simulink model "motorisation_energy_chain"  (R2019b)
settings: Solver=VariableStepAuto  StartTime=0.0  StopTime=10.0  RelTol=1e-3
libraries: simulink x2
settings Model: Creator=ZHOU Jinhan  LastModifiedBy=ZHOU Jinhan

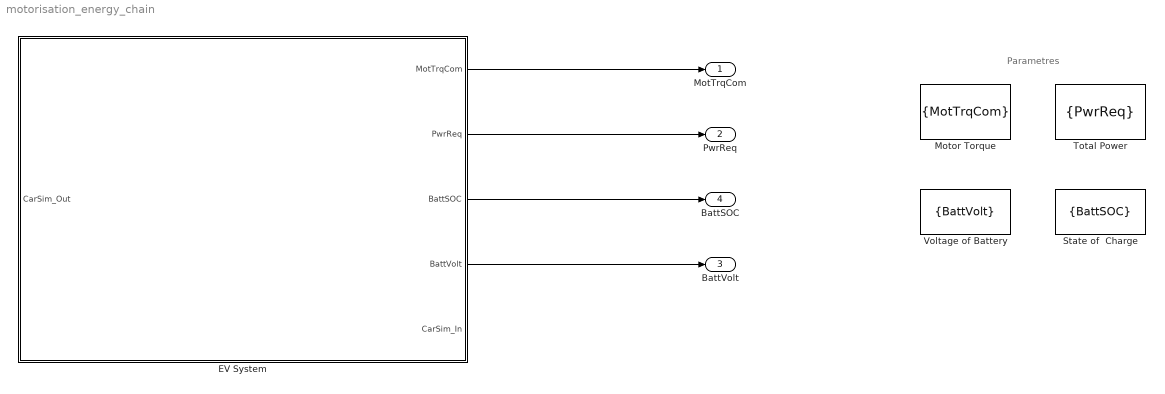
== system motorisation_energy_chain ==
  note: Parametres
  EV System : Subsystem  mask{AmbTem=25, R=0.265}
      mask Display: image('$imagefile'); % Use "Edit Image" on toolstrip to change.
  Motor Torque : GotoTagVisibility  GotoTag=MotTrqCom
  State of  Charge : GotoTagVisibility  GotoTag=BattSOC
  Total Power : GotoTagVisibility  GotoTag=PwrReq
  Voltage of Battery : GotoTagVisibility  GotoTag=BattVolt
  MotTrqCom : Outport
  PwrReq : Outport  Port=2
  BattVolt : Outport  Port=3
  BattSOC : Outport  Port=4
  wires:
  EV System/1(MotTrqCom) -> MotTrqCom/1
  EV System/2(PwrReq) -> PwrReq/1
  EV System/3(BattSOC) -> BattSOC/1
  EV System/4(BattVolt) -> BattVolt/1

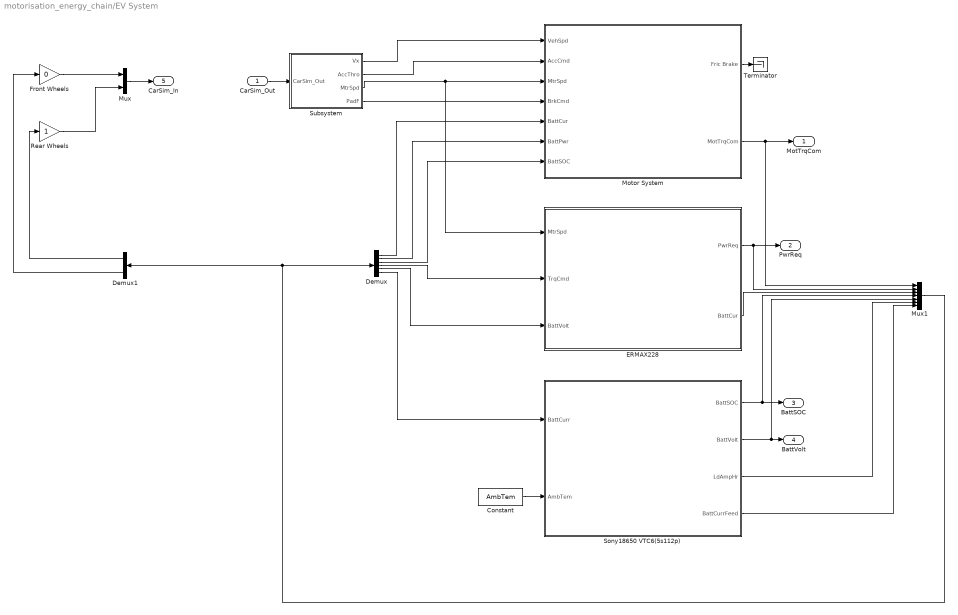
== system motorisation_energy_chain/EV System ==
  CarSim_Out : Inport
  Constant : Constant  Value=AmbTem
  Demux : Demux  Outputs=6
  Demux1 : Demux  Outputs=2
  ERMAX228 : Subsystem  mask{Eff=[83 84 85 84.5 85 84.8 84.59999999999999 84.3 84 83.5 82.8;84 84 86 86 85.8 85.59999999999999 85.59999999999999 85.2 84.5 84 83.3;84 86 87.5 88 88 88 87 86 85 84.5 83.90000000000001;84 87 88.5 90 91 91 90 88 86.2 85.5 84.5;84 87.5 89.5 93.8 93.5 93.8 94.3 91 89.5 86.5 85;84 88 92 94.2 94.5 94.5 95 94 91 91.5 85.8;84 88 92.5 94.59999999999999 95 95.3 95.40000000000001 94.7 92 90.2 85.8;84 88 93 95.59999999999999 96.2 96.3 95.40000000000001 94.90000000000001 93 90.2 85.5;84 88 93 95.8 96.40000000000001 97 95.40000000000001 94.90000000000001 94 90.2 85.8;84 88 92 96 96.59999999999999 97.5 95.40000000000001 94.90000000000001 94 90.2 85.8;84 88 93 95.90000000000001 98 97.5 95.40000000000001 94.90000000000001 94 90.2 85.8;84 88 93 95.90000000000001 97.5 97.5 95.40000000000001 94.90000000000001 94 90.2 85.8;84 88 93 95.59999999999999 97 97.5 95.40000000000001 94.90000000000001 94 90.2 85.8;84 88 93 95.5 96.8 97.3 95.40000000000001 94.90000000000001 94 90.2 85.8;84 86 93 95 96.40000000000001 96.5 95.40000000000001 94.90000000000001 94 90.2 85.8;83.5 85 93 94.8 96.2 96.2 95.40000000000001 94.8 94 90.2 85.8;83.5 84 92 94.59999999999999 95.7 95.7 95.2 94.8 94 90.2 85.8;83.2 83.5 89.5 94.40000000000001 95.2 95.5 95.09999999999999 94.7 94 90.2 85.8;83 83.2 88 94 94.7 95.2 95 94.59999999999999 94 90.2 85.8;82.7 83 86 91 94.3 94.5 94.8 94.59999999999999 94 90.2 85.8;82.5 83.7 85 92 93.8 94.2 94.5 94.5 94 90.2 85.8;82.3 83.40000000000001 84 90 90 93 94.3 94.3 94 90.2 85.8;82 82.7 83 84 85.2 86 94 94 94 90.2 85.8], MtrSpd_sample=[0 1200 1400 1600 1800 2000 2200 2400 2600 2800 3000 3200 3400 3600 3800 4000 4200 4400 4600 4800 5000 6000 7000], MtrTrq_sample=[240 240 240 240 240 240 240 239.1 237.8 236.6 235.7 234.5 233.1 231.6 230.6 228 225.8 222.9 220.6 217.7 216.2 216 216], Spd=[0 250 500 750 1000 1250 1500 1750 2000 2250 2500 2750 3000 3250 3500 3750 4000 4250 4500 4750 5000 5250 5500], Tc=0.02, Trq=[0 25 50 75 100 125 150 175 200 225 250]}
      mask Display: image('$imagefile'); % Use "Edit Image" on toolstrip to change.
  Front Wheels : Gain  Gain=0
  Motor System : Subsystem  mask(DatasheetMotor){Eff=[83 84 85 84.5 85 84.8 84.59999999999999 84.3 84 83.5 82.8;84 84 86 86 85.8 85.59999999999999 85.59999999999999 85.2 84.5 84 83.3;84 86 87.5 88 88 88 87 86 85 84.5 83.90000000000001;84 87 88.5 90 91 91 90 88 86.2 85.5 84.5;84 87.5 89.5 93.8 93.5 93.8 94.3 91 89.5 86.5 85;84 88 92 94.2 94.5 94.5 95 94 91 91.5 85.8;84 88 92.5 94.59999999999999 95 95.3 95.40000000000001 94.7 92 90.2 85.8;84 88 93 95.59999999999999 96.2 96.3 95.40000000000001 94.90000000000001 93 90.2 85.5;84 88 93 95.8 96.40000000000001 97 95.40000000000001 94.90000000000001 94 90.2 85.8;84 88 92 96 96.59999999999999 97.5 95.40000000000001 94.90000000000001 94 90.2 85.8;84 88 93 95.90000000000001 98 97.5 95.40000000000001 94.90000000000001 94 90.2 85.8;84 88 93 95.90000000000001 97.5 97.5 95.40000000000001 94.90000000000001 94 90.2 85.8;84 88 93 95.59999999999999 97 97.5 95.40000000000001 94.90000000000001 94 90.2 85.8;84 88 93 95.5 96.8 97.3 95.40000000000001 94.90000000000001 94 90.2 85.8;84 86 93 95 96.40000000000001 96.5 95.40000000000001 94.90000000000001 94 90.2 85.8;83.5 85 93 94.8 96.2 96.2 95.40000000000001 94.8 94 90.2 85.8;83.5 84 92 94.59999999999999 95.7 95.7 95.2 94.8 94 90.2 85.8;83.2 83.5 89.5 94.40000000000001 95.2 95.5 95.09999999999999 94.7 94 90.2 85.8;83 83.2 88 94 94.7 95.2 95 94.59999999999999 94 90.2 85.8;82.7 83 86 91 94.3 94.5 94.8 94.59999999999999 94 90.2 85.8;82.5 83.7 85 92 93.8 94.2 94.5 94.5 94 90.2 85.8;82.3 83.40000000000001 84 90 90 93 94.3 94.3 94 90.2 85.8;82 82.7 83 84 85.2 86 94 94 94 90.2 85.8], Batt_R1=0.015, MtrSpd_sample=[0 1200 1400 1600 1800 2000 2200 2400 2600 2800 3000 3200 3400 3600 3800 4000 4200 4400 4600 4800 5000 6000 7000], MtrTrq_sample=[240 240 240 240 240 240 240 239.1 237.8 236.6 235.7 234.5 233.1 231.6 230.6 228 225.8 222.9 220.6 217.7 216.2 216 216], Np=5, Ns=112, Pedal_Acc=[0 50 100], Pedal_Spd=[0 250 500 750 1000 1250 1500 1750 2000 2250 2500 2750 3000 3250 3500 3750 4000 4250 4500 4750 5000 5250 5500], Pedal_Trq=[0 0 0 0 0 0 0 0 0 0 0 0 0 0 0 0 0 0 0 0 0 0 0;96 99 102 106 108 112 114 118 120 121 123 126 126 126 126 125 123 120 120 120 115 111 108;240 240 240 240 240 240 240 239.1 237.8 236.6 235.7 234.5 233.1 231.6 230.6 228 225.8 222.9 220.6 217.7 216.2 216 216], PowerLimitBuffer=60000, Power_charge=[89.85599999999999 101.4 102.336 102.96 103.584 104.208 104.52 111.696], Power_discharge=[102.96 102.336 101.4 100.776 100.152 99.84 99.21600000000001 82.67999999999999], SOC_charge=[0 0.15625 0.3125 0.46875 0.625 0.78125 0.9375 1], SOC_discharge=[0 0.15625 0.3125 0.46875 0.625 0.78125 0.9375 1], Spd=[0 250 500 750 1000 1250 1500 1750 2000 2250 2500 2750 3000 3250 3500 3750 4000 4250 4500 4750 5000 5250 5500], Trq=[0 25 50 75 100 125 150 175 200 225 250], Tsb=0.15, Tst=0.1}
      mask Display: image('$imagefile'); % Use "Edit Image" on toolstrip to change.
  Mux : Mux  Inputs=2
  Mux1 : Mux  Inputs=7
  Rear Wheels : Gain
  Sony18650 VTC6(5s112p) : Subsystem  mask{RInt=[18 17 16 15 13 11 10 9.5 9.5 9.5 9.5 9.5;18 16 15 13 11 10 9.5 9 9 9 9 9;18 15 13 11 10 9 8.5 8.5 8.5 8.5 8.5 8.5;18 9 8 8 8 8 8 8 8 8 8 8;18 8 8 8 8 8 8 8 8 8 8 8;18 8 8 8 8 8 8 8 8 8 8 8], BattCapinit=2.85, CapLUTBp=[0 5 10 20 30 40 50 60 70 80 90 100], CapSOCBp=[0 5 10 20 30 40 50 60 70 80 90 100], BattTempBp=[-10 0 10 25 40 45], Em=[3 3.45 3.68 3.74 3.77 3.79 3.82 3.87 3.92 3.98 4.06 4.2], Np=5, Ns=112, CapTem=[-10 0 23 45], CapNom=[2.517894736842106 2.652547368421053 3.120000000000001 3.120000000000001]}
      mask Display: image('$imagefile'); % Use "Edit Image" on toolstrip to change.
  Subsystem : Subsystem
  Terminator : Terminator
  MotTrqCom : Outport
  PwrReq : Outport  Port=2
  BattSOC : Outport  Port=3
  BattVolt : Outport  Port=4
  CarSim_In : Outport  Port=5
  wires:
  Front Wheels/1 -> Mux/1
  Subsystem/1(Vx) -> Motor System/1(VehSpd)
  Sony18650 VTC6(5s112p)/2(BattVolt) -> Mux1/5, BattVolt/1
  Motor System/2(MotTrqCom) -> Mux1/1, MotTrqCom/1
  Subsystem/4(PadF) -> Motor System/4(BrkCmd)
  Motor System/1(Fric Brake) -> Terminator/1
  Subsystem/2(AccThro) -> Motor System/2(AccCmd)
  Subsystem/3(MtrSpd) -> ERMAX228/1(MtrSpd), Motor System/3(MtrSpd)
  ERMAX228/1(PwrReq) -> Mux1/2, PwrReq/1
  Constant/1 -> Sony18650 VTC6(5s112p)/2(AmbTem)
  Sony18650 VTC6(5s112p)/1(BattSOC) -> Mux1/4, BattSOC/1
  CarSim_Out/1 -> Subsystem/1(CarSim_Out)
  Mux/1 -> CarSim_In/1
  Rear Wheels/1 -> Mux/2
  ERMAX228/2(BattCur) -> Mux1/3
  Sony18650 VTC6(5s112p)/3(LdAmpHr) -> Mux1/6
  Sony18650 VTC6(5s112p)/4(BattCurrFeed) -> Mux1/7
  Mux1/1 -> Demux/1, Demux1/1
  Demux/1 -> Motor System/5(BattCur)
  Demux/2 -> Motor System/6(BattPwr)
  Demux/3 -> Motor System/7(BattSOC)
  Demux/4 -> ERMAX228/2(TrqCmd)
  Demux/5 -> ERMAX228/3(BattVolt)
  Demux/6 -> Sony18650 VTC6(5s112p)/1(BattCurr)
  Demux1/1 -> Rear Wheels/1
  Demux1/2 -> Front Wheels/1

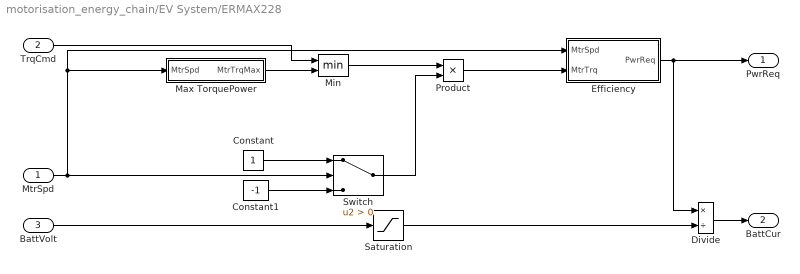
== system motorisation_energy_chain/EV System/ERMAX228 ==
  MtrSpd : Inport
  TrqCmd : Inport  Port=2
  BattVolt : Inport  Port=3
  Constant : Constant
  Constant1 : Constant  Value=-1
  Divide : Product  Inputs=*/
  Efficiency : Subsystem
  Max TorquePower : Subsystem
  Min : MinMax  Inputs=2
  Product : Product
  Saturation : Saturate  UpperLimit=Inf  LowerLimit=0.001
  Switch : Switch  Criteria=u2 > Threshold
  PwrReq : Outport
  BattCur : Outport  Port=2
  wires:
  Saturation/1 -> Divide/2
  BattVolt/1 -> Saturation/1
  Divide/1 -> BattCur/1
  Switch/1 -> Product/2
  TrqCmd/1 -> Min/1
  Max TorquePower/1(MtrTrqMax) -> Min/2
  Product/1 -> Efficiency/2(MtrTrq)
  Min/1 -> Product/1
  Constant/1 -> Switch/1
  Constant1/1 -> Switch/3
  Efficiency/1(PwrReq) -> PwrReq/1, Divide/1
  MtrSpd/1 -> Switch/2, Max TorquePower/1(MtrSpd), Efficiency/1(MtrSpd)

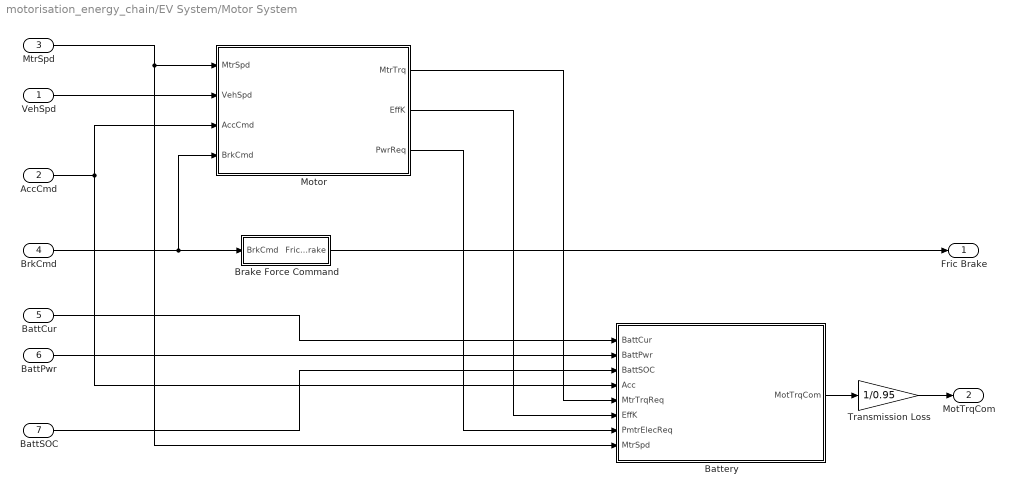
== system motorisation_energy_chain/EV System/Motor System ==
  VehSpd : Inport
  AccCmd : Inport  Port=2
  MtrSpd : Inport  Port=3
  BrkCmd : Inport  Port=4
  BattCur : Inport  Port=5
  BattPwr : Inport  Port=6
  BattSOC : Inport  Port=7
  Battery : Subsystem
  Brake Force Command : Subsystem
  Motor : Subsystem  mask{R=0.265}
  Transmission Loss : Gain  Gain=1/0.95
  Fric Brake : Outport
  MotTrqCom : Outport  Port=2
  wires:
  Battery/1(MotTrqCom) -> Transmission Loss/1
  BattSOC/1 -> Battery/3(BattSOC)
  BattPwr/1 -> Battery/2(BattPwr)
  VehSpd/1 -> Motor/2(VehSpd)
  Motor/1(MtrTrq) -> Battery/5(MtrTrqReq)
  AccCmd/1 -> Battery/4(Acc), Motor/3(AccCmd)
  BattCur/1 -> Battery/1(BattCur)
  BrkCmd/1 -> Brake Force Command/1(BrkCmd), Motor/4(BrkCmd)
  Motor/3(PwrReq) -> Battery/7(PmtrElecReq)
  MtrSpd/1 -> Motor/1(MtrSpd), Battery/8(MtrSpd)
  Brake Force Command/1(Fric Brake) -> Fric Brake/1
  Motor/2(EffK) -> Battery/6(EffK)
  Transmission Loss/1 -> MotTrqCom/1

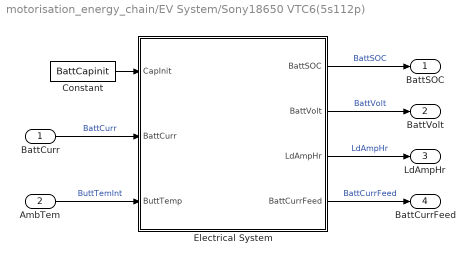
== system motorisation_energy_chain/EV System/Sony18650 VTC6(5s112p) ==
  BattCurr : Inport
  AmbTem : Inport  Port=2
  Constant : Constant  Value=BattCapinit
  Electrical System : Subsystem
  BattSOC : Outport
  BattVolt : Outport  Port=2
  LdAmpHr : Outport  Port=3
  BattCurrFeed : Outport  Port=4
  wires:
  AmbTem/1 -> Electrical System/3(ButtTemp)  "ButtTemInt"
  Electrical System/4(BattCurrFeed) -> BattCurrFeed/1  "BattCurrFeed"
  Electrical System/1(BattSOC) -> BattSOC/1  "BattSOC"
  Electrical System/3(LdAmpHr) -> LdAmpHr/1  "LdAmpHr"
  BattCurr/1 -> Electrical System/2(BattCurr)  "BattCurr"
  Electrical System/2(BattVolt) -> BattVolt/1  "BattVolt"
  Constant/1 -> Electrical System/1(CapInit)

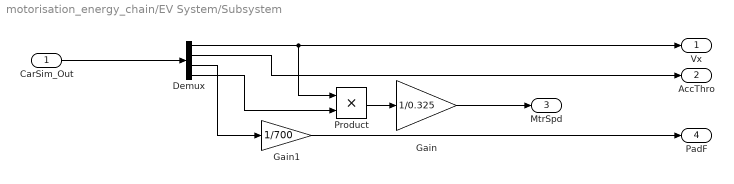
== system motorisation_energy_chain/EV System/Subsystem ==
  CarSim_Out : Inport
  Demux : Demux
  Gain : Gain  Gain=1/0.325
  Gain1 : Gain  Gain=1/700
  Product : Product
  Vx : Outport
  AccThro : Outport  Port=2
  MtrSpd : Outport  Port=3
  PadF : Outport  Port=4
  wires:
  Demux/2 -> AccThro/1
  Demux/3 -> Gain1/1
  Product/1 -> Gain/1
  CarSim_Out/1 -> Demux/1
  Demux/1 -> Vx/1, Product/1
  Demux/4 -> Product/2
  Gain/1 -> MtrSpd/1
  Gain1/1 -> PadF/1

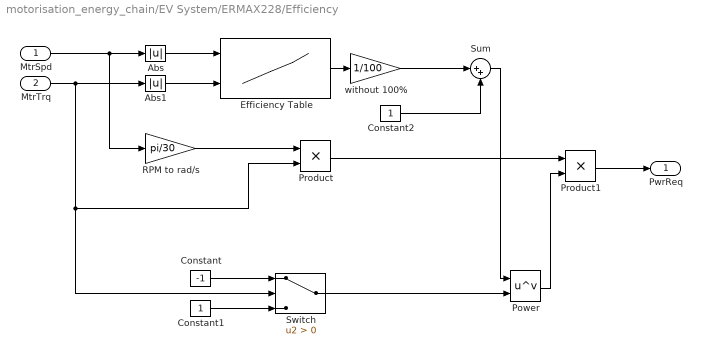
== system motorisation_energy_chain/EV System/ERMAX228/Efficiency ==
  MtrSpd : Inport
  MtrTrq : Inport  Port=2
  Abs : Abs
  Abs1 : Abs
  Constant : Constant  Value=-1
  Constant1 : Constant
  Constant2 : Constant
  Efficiency Table : Lookup_n-D  LookupTableObject=Efficiency  BreakpointsForDimension1=Spd  BreakpointsForDimension2=Trq  Table=Eff  InterpMethod=Linear Lagrange  InternalRulePriority=Speed  RndMeth=Simplest  InputSameDT=on
  Power : Math  Operator=pow  SignedPower=off  SaturateOnIntegerOverflow=on
  Product : Product
  Product1 : Product
  RPM to rad/s : Gain  Gain=pi/30
  Sum : Sum  Inputs=|++
  Switch : Switch  Criteria=u2 > Threshold
  without 100% : Gain  Gain=1/100
  PwrReq : Outport
  wires:
  Product1/1 -> PwrReq/1
  Power/1 -> Product1/2
  Product/1 -> Product1/1
  Constant2/1 -> Sum/2
  RPM to rad/s/1 -> Product/1
  Switch/1 -> Power/2
  Constant1/1 -> Switch/3
  Constant/1 -> Switch/1
  without 100%/1 -> Sum/1
  Abs1/1 -> Efficiency Table/2
  Abs/1 -> Efficiency Table/1
  Sum/1 -> Power/1
  Efficiency Table/1 -> without 100%/1
  MtrTrq/1 -> Abs1/1, Product/2, Switch/2
  MtrSpd/1 -> Abs/1, RPM to rad/s/1

== system motorisation_energy_chain/EV System/ERMAX228/Max TorquePower ==
  MtrSpd : Inport
  Abs : Abs
  MaxTrq(|MtrSpd|) : Lookup_n-D  NumberOfTableDimensions=1  BreakpointsForDimension1=MtrSpd_sample  Table=MtrTrq_sample  InterpMethod=Linear Lagrange  InternalRulePriority=Speed  RndMeth=Simplest  InputSameDT=on
  Signal Conversion : SignalConversion  OverrideOpt=off
  MtrTrqMax : Outport
  wires:
  MtrSpd/1 -> Abs/1
  Signal Conversion/1 -> MtrTrqMax/1
  MaxTrq(|MtrSpd|)/1 -> Signal Conversion/1
  Abs/1 -> MaxTrq(|MtrSpd|)/1

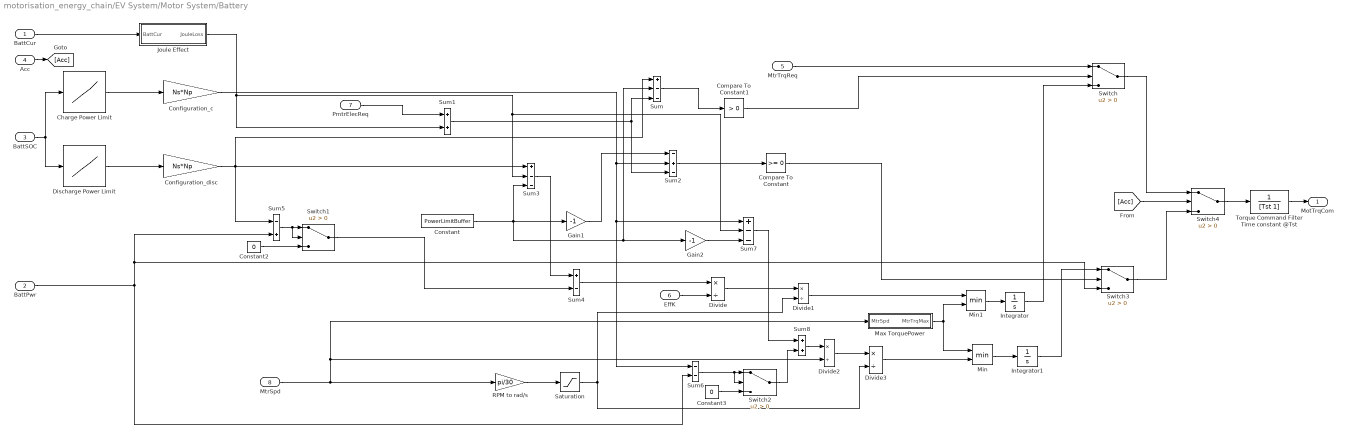
== system motorisation_energy_chain/EV System/Motor System/Battery ==
  BattCur : Inport
  BattPwr : Inport  Port=2
  BattSOC : Inport  Port=3
  Acc : Inport  Port=4
  MtrTrqReq : Inport  Port=5
  EffK : Inport  Port=6
  PmtrElecReq : Inport  Port=7
  MtrSpd : Inport  Port=8
  Charge Power Limit : Lookup_n-D  NumberOfTableDimensions=1  BreakpointsForDimension1=SOC_charge  Table=Power_charge  InterpMethod=Linear Lagrange  InternalRulePriority=Speed  RndMeth=Simplest  InputSameDT=on
  Compare To Constant : simulink/Logic and Bit Operations/Compare To Constant  relop=>=  const=0  OutDataTypeStr=boolean
  Compare To Constant1 : simulink/Logic and Bit Operations/Compare To Constant  relop=>  const=0  OutDataTypeStr=boolean
  Configuration_c : Gain  Gain=Ns*Np
  Configuration_disc : Gain  Gain=Ns*Np
  Constant : Constant  Value=PowerLimitBuffer
  Constant2 : Constant  Value=0
  Constant3 : Constant  Value=0
  Discharge Power Limit : Lookup_n-D  NumberOfTableDimensions=1  BreakpointsForDimension1=SOC_discharge  Table=Power_discharge  InterpMethod=Linear Lagrange  InternalRulePriority=Speed  RndMeth=Simplest  InputSameDT=on
  Divide{,1..3} (4 alike) : Product  Inputs=*/
  Gain1 : Gain  Gain=-1
  Gain2 : Gain  Gain=-1
  Integrator : Integrator
  Integrator1 : Integrator
  Joule Effect : Subsystem
  Max TorquePower : Subsystem
  Min : MinMax  Inputs=2
  Min1 : MinMax  Inputs=2
  RPM to rad/s : Gain  Gain=pi/30
  Saturation : Saturate  UpperLimit=Inf  LowerLimit=0.0001
  Sum : Sum  Inputs=+--
  Sum1 : Sum
  Sum2 : Sum  Inputs=-+-
  Sum3 : Sum  Inputs=+--
  Sum4 : Sum  Inputs=+-
  Sum5 : Sum  Inputs=-+
  Sum6 : Sum  Inputs=--
  Sum7 : Sum  Inputs=+--
  Sum8 : Sum
  Switch{,1..4} (5 alike) : Switch  Criteria=u2 > Threshold
  Torque Command Filter Time constant @Tst : TransferFcn  Denominator=[Tst 1]
  MotTrqCom : Outport
  wires:
  Charge Power Limit/1 -> Configuration_c/1
  Discharge Power Limit/1 -> Configuration_disc/1
  Configuration_disc/1 -> Sum5/1, Sum3/1, Sum/1
  Configuration_c/1 -> Sum2/2, Sum7/1, Sum6/1
  Gain2/1 -> Sum7/3
  BattCur/1 -> Joule Effect/1(BattCur)
  Joule Effect/1(JouleLoss) -> Sum1/2, Sum7/2, Sum3/2
  Divide3/1 -> Min/2
  Divide1/1 -> Min1/1
  Max TorquePower/1(MtrTrqMax) -> Min1/2, Min/1
  Min1/1 -> Integrator/1
  Acc/1 -> [Acc]
  RPM to rad/s/1 -> Saturation/1
  Min/1 -> Integrator1/1
  PmtrElecReq/1 -> Sum1/1
  Switch4/1 -> Torque Command Filter Time constant @Tst/1
  Constant3/1 -> Switch2/3
  Sum2/1 -> Compare To Constant/1
  Sum6/1 -> Switch2/1, Switch2/2
  Switch3/1 -> Switch4/3
  Integrator1/1 -> Switch3/1
  Sum5/1 -> Switch1/1, Switch1/2
  Sum4/1 -> Divide/1
  Divide/1 -> Divide1/1
  Sum3/1 -> Sum4/1
  Gain1/1 -> Sum2/1
  Sum8/1 -> Divide2/1
  Switch1/1 -> Sum4/2
  EffK/1 -> Divide/2
  Compare To Constant1/1 -> Switch/2
  Constant2/1 -> Switch1/3
  Compare To Constant/1 -> Switch3/2
  Sum/1 -> Compare To Constant1/1
  Switch/1 -> Switch4/1
  Divide2/1 -> Divide3/1
  BattSOC/1 -> Charge Power Limit/1, Discharge Power Limit/1
  [Acc] -> Switch4/2
  Sum1/1 -> Sum/3, Sum2/3
  Torque Command Filter Time constant @Tst/1 -> MotTrqCom/1
  Saturation/1 -> Divide1/2, Divide3/2
  BattPwr/1 -> Switch3/3, Sum5/2, Sum6/2
  Switch2/1 -> Sum8/2
  Sum7/1 -> Sum8/1
  Constant/1 -> Gain1/1, Gain2/1, Sum/2, Sum3/3
  MtrSpd/1 -> RPM to rad/s/1, Divide2/2, Max TorquePower/1(MtrSpd)
  Integrator/1 -> Switch/3
  MtrTrqReq/1 -> Switch/1

== system motorisation_energy_chain/EV System/Motor System/Brake Force Command ==
  BrkCmd : Inport
  Brake Command Filter Time constant @Tsb : TransferFcn  Denominator=[Tsb 1]
  Friction Brake Command : Lookup_n-D  NumberOfTableDimensions=1  BreakpointsForDimension1=[0 0.1 0.2 0.4 0.6 0.8 1]  Table=[0 0 0.2 0.4 0.6 0.8 1]*60  InternalRulePriority=Speed  RndMeth=Simplest  InputSameDT=on
  Fric Brake : Outport
  wires:
  Friction Brake Command/1 -> Brake Command Filter Time constant @Tsb/1
  Brake Command Filter Time constant @Tsb/1 -> Fric Brake/1
  BrkCmd/1 -> Friction Brake Command/1

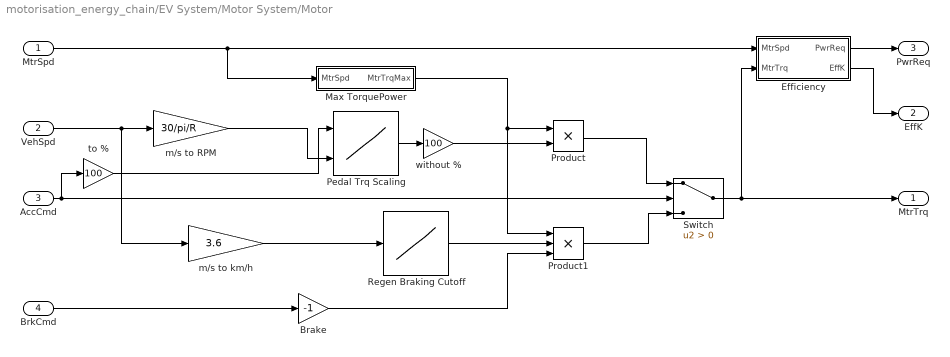
== system motorisation_energy_chain/EV System/Motor System/Motor ==
  MtrSpd : Inport
  VehSpd : Inport  Port=2
  AccCmd : Inport  Port=3
  BrkCmd : Inport  Port=4
  Brake : Gain  Gain=-1
  Efficiency : Subsystem
  Max TorquePower : Subsystem
  Pedal Trq Scaling : Lookup_n-D  BreakpointsForDimension1=Pedal_Acc  BreakpointsForDimension2=Pedal_Spd  Table=Pedal_Trq  InterpMethod=Linear Lagrange  InternalRulePriority=Speed  RndMeth=Simplest  InputSameDT=on
  Product : Product
  Product1 : Product  Inputs=3
  Regen Braking Cutoff : Lookup_n-D  NumberOfTableDimensions=1  BreakpointsForDimension1=[0.5 1]  BeginIndexSearchUsingPreviousIndexResult=on  Table=[0 1]  ExtrapMethod=Clip  InternalRulePriority=Speed  RndMeth=Simplest  InputSameDT=on
  Switch : Switch  Criteria=u2 > Threshold
  m/s to RPM : Gain  Gain=30/pi/R
  m/s to km/h : Gain  Gain=3.6
  to % : Gain  Gain=100
  without % : Gain  Gain=100
  MtrTrq : Outport
  EffK : Outport  Port=2
  PwrReq : Outport  Port=3
  wires:
  to %/1 -> Pedal Trq Scaling/1
  Efficiency/2(EffK) -> EffK/1
  Brake/1 -> Product1/3
  Regen Braking Cutoff/1 -> Product1/2
  Switch/1 -> Efficiency/2(MtrTrq), MtrTrq/1
  Product1/1 -> Switch/3
  BrkCmd/1 -> Brake/1
  Product/1 -> Switch/1
  Max TorquePower/1(MtrTrqMax) -> Product/1, Product1/1
  without %/1 -> Product/2
  Pedal Trq Scaling/1 -> without %/1
  AccCmd/1 -> Switch/2, to %/1
  Efficiency/1(PwrReq) -> PwrReq/1
  MtrSpd/1 -> Max TorquePower/1(MtrSpd), Efficiency/1(MtrSpd)
  m/s to RPM/1 -> Pedal Trq Scaling/2
  VehSpd/1 -> m/s to km/h/1, m/s to RPM/1
  m/s to km/h/1 -> Regen Braking Cutoff/1

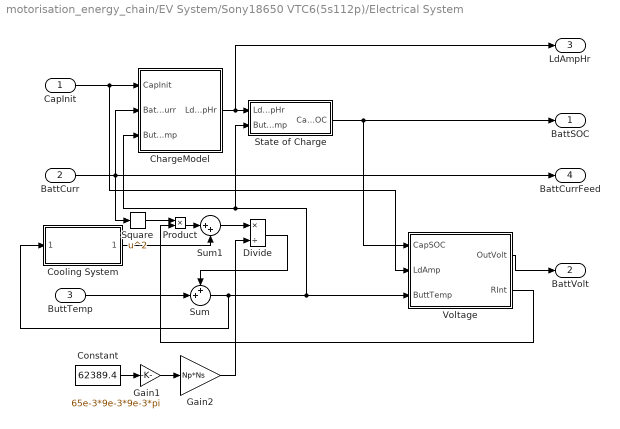
== system motorisation_energy_chain/EV System/Sony18650 VTC6(5s112p)/Electrical System ==
  CapInit : Inport
  BattCurr : Inport  Port=2
  ButtTemp : Inport  Port=3
  ChargeModel : Subsystem
  Constant : Constant  Value=62389.4
  Cooling System : Subsystem
  Divide : Product  Inputs=*/
  Gain1 : Gain  Gain=65e-3*9e-3*9e-3*pi
  Gain2 : Gain  Gain=Np*Ns
  Product : Product
  Square : Math  Operator=square  SignedPower=off  SaturateOnIntegerOverflow=on
  State of Charge : Subsystem
  Sum : Sum  Inputs=++|
  Sum1 : Sum  Inputs=|++
  Voltage : Subsystem
  BattSOC : Outport
  BattVolt : Outport  Port=2
  LdAmpHr : Outport  Port=3
  BattCurrFeed : Outport  Port=4
  wires:
  Voltage/1(OutVolt) -> BattVolt/1
  BattCurr/1 -> ChargeModel/2(BattCurr), Square/1, BattCurrFeed/1
  CapInit/1 -> Voltage/2(LdAmp), ChargeModel/1(CapInit)
  State of Charge/1(CapSOC) -> Voltage/1(CapSOC), BattSOC/1
  ChargeModel/1(LdAmpHr) -> State of Charge/1(LdAmpHr), LdAmpHr/1
  ButtTemp/1 -> Sum/2
  Sum/1 -> Cooling System/1(BattVolt), Voltage/3(ButtTemp), State of Charge/2(ButtTemp), ChargeModel/3(ButtTemp)
  Voltage/2(RInt) -> Product/2
  Square/1 -> Product/1
  Product/1 -> Sum1/1
  Sum1/1 -> Divide/1
  Gain2/1 -> Divide/2
  Divide/1 -> Sum/1
  Constant/1 -> Gain1/1
  Gain1/1 -> Gain2/1
  Cooling System/1(CoolTem) -> Sum1/2

== system motorisation_energy_chain/EV System/Motor System/Battery/Joule Effect ==
  BattCur : Inport
  Configuration : Gain  Gain=Ns/Np
  Gain : Gain  Gain=Batt_R1
  Square : Math  Operator=square  SignedPower=off  SaturateOnIntegerOverflow=on
  JouleLoss : Outport
  wires:
  Configuration/1 -> JouleLoss/1
  Gain/1 -> Configuration/1
  BattCur/1 -> Square/1
  Square/1 -> Gain/1

== system motorisation_energy_chain/EV System/Motor System/Battery/Max TorquePower ==
  MtrSpd : Inport
  Abs : Abs
  MaxTrq(|MtrSpd|) : Lookup_n-D  NumberOfTableDimensions=1  BreakpointsForDimension1=MtrSpd_sample  Table=MtrTrq_sample  InterpMethod=Linear Lagrange  InternalRulePriority=Speed  RndMeth=Simplest  InputSameDT=on
  Signal Conversion : SignalConversion  OverrideOpt=off
  MtrTrqMax : Outport
  wires:
  MtrSpd/1 -> Abs/1
  Signal Conversion/1 -> MtrTrqMax/1
  MaxTrq(|MtrSpd|)/1 -> Signal Conversion/1
  Abs/1 -> MaxTrq(|MtrSpd|)/1

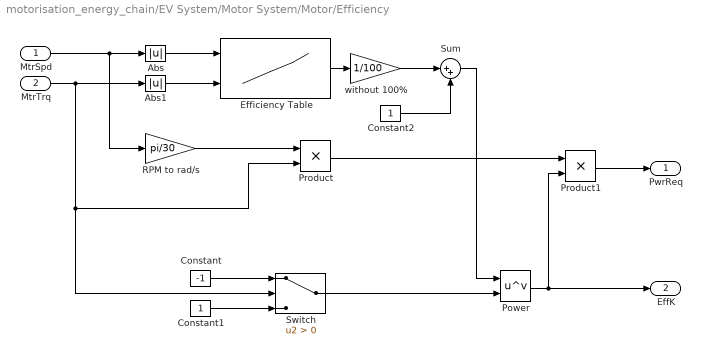
== system motorisation_energy_chain/EV System/Motor System/Motor/Efficiency ==
  MtrSpd : Inport
  MtrTrq : Inport  Port=2
  Abs : Abs
  Abs1 : Abs
  Constant : Constant  Value=-1
  Constant1 : Constant
  Constant2 : Constant
  Efficiency Table : Lookup_n-D  LookupTableObject=Efficiency  BreakpointsForDimension1=Spd  BreakpointsForDimension2=Trq  Table=Eff  InterpMethod=Linear Lagrange  InternalRulePriority=Speed  RndMeth=Simplest  InputSameDT=on
  Power : Math  Operator=pow  SignedPower=off  SaturateOnIntegerOverflow=on
  Product : Product
  Product1 : Product
  RPM to rad/s : Gain  Gain=pi/30
  Sum : Sum  Inputs=|++
  Switch : Switch  Criteria=u2 > Threshold
  without 100% : Gain  Gain=1/100
  PwrReq : Outport
  EffK : Outport  Port=2
  wires:
  Product1/1 -> PwrReq/1
  Power/1 -> EffK/1, Product1/2
  Product/1 -> Product1/1
  Constant2/1 -> Sum/2
  RPM to rad/s/1 -> Product/1
  Switch/1 -> Power/2
  Constant1/1 -> Switch/3
  Constant/1 -> Switch/1
  without 100%/1 -> Sum/1
  Abs1/1 -> Efficiency Table/2
  Abs/1 -> Efficiency Table/1
  Sum/1 -> Power/1
  Efficiency Table/1 -> without 100%/1
  MtrTrq/1 -> Abs1/1, Product/2, Switch/2
  MtrSpd/1 -> Abs/1, RPM to rad/s/1

== system motorisation_energy_chain/EV System/Motor System/Motor/Max TorquePower ==
  MtrSpd : Inport
  Abs : Abs
  MaxTrq(|MtrSpd|) : Lookup_n-D  NumberOfTableDimensions=1  BreakpointsForDimension1=MtrSpd_sample  Table=MtrTrq_sample  InterpMethod=Linear Lagrange  InternalRulePriority=Speed  RndMeth=Simplest  InputSameDT=on
  Signal Conversion : SignalConversion  OverrideOpt=off
  MtrTrqMax : Outport
  wires:
  MtrSpd/1 -> Abs/1
  Signal Conversion/1 -> MtrTrqMax/1
  MaxTrq(|MtrSpd|)/1 -> Signal Conversion/1
  Abs/1 -> MaxTrq(|MtrSpd|)/1

== system motorisation_energy_chain/EV System/Sony18650 VTC6(5s112p)/Electrical System/ChargeModel ==
  CapInit : Inport
  BattCurr : Inport  Port=2
  ButtTemp : Inport  Port=3
  BattChargeMax : Lookup_n-D  NumberOfTableDimensions=1  BreakpointsForDimension1=CapTem  Table=CapNom  InterpMethod=Linear Lagrange  InternalRulePriority=Speed  RndMeth=Simplest  InputSameDT=on
  Gain : Gain  Gain=-1/(Np*3600)
  Integrator Limited : Integrator  InitialConditionSource=external  LimitOutput=on  UpperSaturationLimit=1  LowerSaturationLimit=0
  Switch : Switch  Criteria=u2 > Threshold
  LdAmpHr : Outport
  wires:
  ButtTemp/1 -> BattChargeMax/1
  Switch/1 -> Integrator Limited/2
  Integrator Limited/1 -> LdAmpHr/1
  CapInit/1 -> Switch/3, Switch/2
  Gain/1 -> Integrator Limited/1
  BattCurr/1 -> Gain/1
  BattChargeMax/1 -> Switch/1

== system motorisation_energy_chain/EV System/Sony18650 VTC6(5s112p)/Electrical System/Cooling System ==
  BattVolt : Inport
  AmbTem : Constant  Value=25
  Fans Nombre : Gain  Gain=2
  Gain : Gain  Gain=34.61*1.003*4.2
  Sum2 : Sum  Inputs=+-|
  CoolTem : Outport
  wires:
  Gain/1 -> Fans Nombre/1
  Sum2/1 -> Gain/1
  AmbTem/1 -> Sum2/2
  BattVolt/1 -> Sum2/1
  Fans Nombre/1 -> CoolTem/1

== system motorisation_energy_chain/EV System/Sony18650 VTC6(5s112p)/Electrical System/State of Charge ==
  LdAmpHr : Inport
  ButtTemp : Inport  Port=2
  BattChargeMax : Lookup_n-D  NumberOfTableDimensions=1  BreakpointsForDimension1=CapTem  Table=CapNom  InterpMethod=Linear Lagrange  InternalRulePriority=Speed  RndMeth=Simplest  InputSameDT=on
  Divide : Product  Inputs=*/
  CapSOC : Outport
  wires:
  ButtTemp/1 -> BattChargeMax/1
  Divide/1 -> CapSOC/1
  LdAmpHr/1 -> Divide/1
  BattChargeMax/1 -> Divide/2

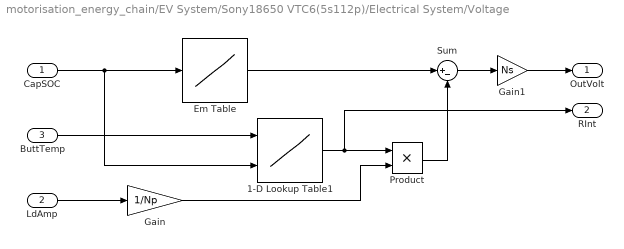
== system motorisation_energy_chain/EV System/Sony18650 VTC6(5s112p)/Electrical System/Voltage ==
  CapSOC : Inport
  LdAmp : Inport  Port=2
  ButtTemp : Inport  Port=3
  1-D Lookup Table1 : Lookup_n-D  BreakpointsForDimension1=BattTempBp  BreakpointsForDimension2=CapSOCBp  Table=RInt.*1e-3  InternalRulePriority=Speed  RndMeth=Simplest  InputSameDT=on
  Em Table : Lookup_n-D  NumberOfTableDimensions=1  BreakpointsForDimension1=CapLUTBp  Table=Em  InterpMethod=Linear Lagrange  InternalRulePriority=Speed  RndMeth=Simplest  InputSameDT=on
  Gain : Gain  Gain=1/Np
  Gain1 : Gain  Gain=Ns
  Product : Product
  Sum : Sum  Inputs=|+-
  OutVolt : Outport
  RInt : Outport  Port=2
  wires:
  1-D Lookup Table1/1 -> RInt/1, Product/1
  Gain1/1 -> OutVolt/1
  CapSOC/1 -> Em Table/1, 1-D Lookup Table1/2
  LdAmp/1 -> Gain/1
  Product/1 -> Sum/2
  Gain/1 -> Product/2
  Sum/1 -> Gain1/1
  Em Table/1 -> Sum/1
  ButtTemp/1 -> 1-D Lookup Table1/1
